simulink model "closed_loop"  (R2019a)
settings: Solver=FixedStepAuto  StartTime=0.0  StopTime=20  FixedStep=1/100  RelTol=1e-3  AbsTol=1e-3
model workspace: external: MAT-File params.mat (data not in the file)
values from neighbouring files (symbols this model uses):
  An = double(subs(A, [x;ctrl] , [x_lin; u_lin] ))    [linearization.m]
  b = 2.75E-11    (= 2.75e-11)    [linearization.m]    (also in main.m)
  Bn = double(subs(B, [x;ctrl] , [x_lin; u_lin] ))    [linearization.m]
  Cn = eye(size(x,1))    [linearization.m]
  Dn = zeros(size(x,1),4)    [linearization.m]
  g = 9.81    [linearization.m]    (also in main.m)
  k = 1E-9    (= 1e-09)    [linearization.m]    (also in main.m)
  m = 0.027    [linearization.m]    (also in main.m)
  ref_base_thrust = 0    [main.m]
  ref_roll_pitch_yawrate = [0 0 0]'    [main.m]
  u_lin = repmat(0.027*g/4, [4 1])    [main.m]
  x0 = [0 0 0  0 0 0  deg2rad(20) deg2rad(20) deg2rad(0) 0 0 0]'    [main.m]
  x_lin = zeros(12,1)    [main.m]
libraries: nesl_utility x9
settings Model: Creator=Jocke  LastModifiedBy=lucas
settings SolverCC: AutoScaleAbsTol=off
settings DataIOCC: ReturnWorkspaceOutputs=off
settings OptimizationCC: UseDivisionForNetSlopeComputation=on
settings DebuggingCC: ArithmeticOperatorsInVariantConditions=warning
settings SFSimCC: SimUseLocalCustomCode=off
settings RTWCC: RTWUseLocalCustomCode=off
settings CodeAppCC: StateflowObjectComments=on
settings SimscapeCC: SimscapeNormalizeSystem=off  SimscapeLogType=all  SimscapeLogDataHistory=10000

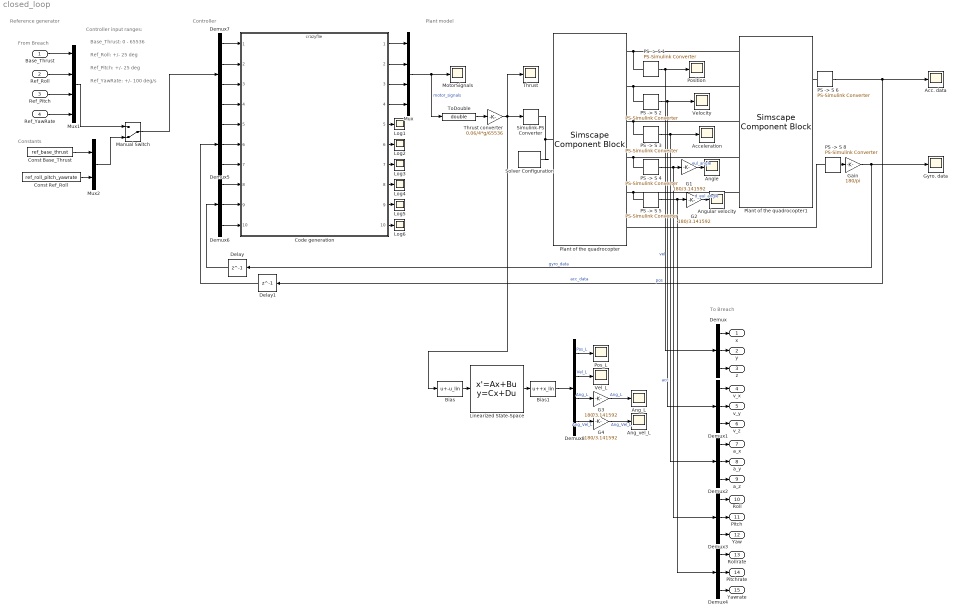
== system closed_loop ==
  note: To Breach
  note: From Breach
  note: Plant model
  note: Controller
  note: Constants
  note: Reference generator
  note: Ref_Roll: +/- 25 deg
  note: Base_Thrust: 0 - 65536
  note: Ref_Pitch: +/- 25 deg
  note: Ref_YawRate: +/- 100 deg/s
  note: Controller input ranges:
  Base_Thrust : Inport  OutDataTypeStr=double
  Ref_Roll : Inport  Port=2  OutDataTypeStr=double
  Ref_Pitch : Inport  Port=3  OutDataTypeStr=double
  Ref_YawRate : Inport  Port=4  OutDataTypeStr=double
  Acc. data : Scope
  Acceleration : Scope
  Ang_L : Scope
  Ang_vel_L : Scope
  Angle : Scope
  Angular velocity : Scope
  Bias : Bias  Bias=-u_lin
  Bias1 : Bias  Bias=+x_lin
  Code generation : ModelReference  ModelNameDialog=crazyflie.slx  SimulationMode=Normal  ModelReferenceVersion=1.283
  Const Base_Thrust : Constant  Value=ref_base_thrust
  Const Ref_Roll : Constant  Value=ref_roll_pitch_yawrate
  Delay : Delay  DelayLength=1
  Delay1 : Delay  DelayLength=1
  Demux{,1..6} (7 alike) : Demux  Outputs=3
  Demux7 : Demux
  Demux8 : Demux
  G{1..4} (4 alike) : Gain  Gain=180/3.141592
  Gain : Gain  Gain=180/pi
  Gyro. data : Scope
  Linearized State-Space : StateSpace  A=An  B=Bn  C=Cn  D=Dn  InitialCondition=x0
  Log{1..6} (6 alike) : Scope
  Manual Switch : ManualSwitch  CurrentSetting=0
  MotorSignals : Scope
  Mux : Mux
  Mux1 : Mux
  Mux2 : Mux  Inputs=2
  PS -> S {1..6,8} (7 alike) : nesl_utility/PS-Simulink Converter  PhysicalDomain=network_engine_domain  SubClassName=ps_output  LeftPortType=input  RightPortType=output  PseudoPeriodic=off  Frequencies=[]  Unit=1  AffineConversion=off
  Plant of the quadrocopter : SimscapeComponentBlock  SourceFile=plant  ComponentPath=plant  ComponentVariants=plant  ComponentVariantNames=plant  ClassName=plant  SchemaVersion=1  m=m kg  g=g m/s^2  d=d m  k=k s^2*N/rad^2  b=b N*m/(rad/s)^2  x0=x0
      settings: CopyFcn=simscape.engine.sli.internal.componentblockcallback(gcbh,'COPY')  PreCopyFcn=simscape.engine.sli.internal.componentblockcallback(gcbh,'PRECOPY')  PreDeleteFcn=simscape.engine.sli.internal.componentblockcallback(gcbh,'PREDELETE')
      mask Type: Plant of quadrocopter
  Plant of the quadrocopter1 : SimscapeComponentBlock  SourceFile=sensors  ComponentPath=sensors  ComponentVariants=sensors  ComponentVariantNames=sensors  ClassName=sensors  SchemaVersion=1
      settings: CopyFcn=simscape.engine.sli.internal.componentblockcallback(gcbh,'COPY')  PreCopyFcn=simscape.engine.sli.internal.componentblockcallback(gcbh,'PRECOPY')  PreDeleteFcn=simscape.engine.sli.internal.componentblockcallback(gcbh,'PREDELETE')
      mask Type: Plant of quadrocopter
  Pos_L : Scope
  Position : Scope
  Simulink-PS Converter : nesl_utility/Simulink-PS Converter  PhysicalDomain=network_engine_domain  SubClassName=ps_input  LeftPortType=input  RightPortType=output  PseudoPeriodic=off  Frequencies=[]  NoiseDistribution=none  NoiseParameters=[]  Unit=1  AffineConversion=off  FilteringAndDerivatives=zero  SimscapeFilterOrder=1  InputFilterTimeConstant=0.001  UdotUserProvided=1
  Solver Configuration : nesl_utility/Solver Configuration  PhysicalDomain=network_engine_domain  SubClassName=solver  LeftPortType=input  RightPortType=generic  Tones=[]  Harmonics=[]  SimulateNoise=off  Profile=off  UseLocalSampling=off  EnableSwitchedLinearOptims=on  FrequencyDomain=off  UseCCode=off  RelTol=0.001  AbsTol=1e-06  MinStep=1e-09  ToWorkspace=off  RevertToSquareIcSolve=off  NumHomotopyIterations=100  PhasorMode=off  PhasorModeNumHarmonics=1  DoDC=off  ResidualTolerance=1e-09  UseLocalSolver=off  LocalSolverChoice=NE_BACKWARD_EULER_ADVANCER  LocalSolverSampleTime=0.001  DoFixedCost=off  MaxNonlinIter=3  MaxModeIter=2  LinearAlgebra=Sparse  EquationFormulation=NE_TIME_EF  DelaysMemoryBudget=1024  AutomaticFiltering=on  FilteringTimeConstant=0.001  PartitionStorageMethod=AS_NEEDED  PartitionMemoryBudget=1024  PartitionMethod=FAST
  Thrust : Scope
  Thrust converter : Gain  Gain=0.06/4*g/65536
  ToDouble : DataTypeConversion  OutDataTypeStr=double  RndMeth=Round  SaturateOnIntegerOverflow=on
  Vel_L : Scope
  Velocity : Scope
  x : Outport
  y : Outport  Port=2
  z : Outport  Port=3
  v_x : Outport  Port=4
  v_y : Outport  Port=5
  v_z : Outport  Port=6
  a_x : Outport  Port=7
  a_y : Outport  Port=8
  a_z : Outport  Port=9
  Roll : Outport  Port=10
  Pitch : Outport  Port=11
  Yaw : Outport  Port=12
  Rollrate : Outport  Port=13
  Pitchrate : Outport  Port=14
  Yawrate : Outport  Port=15
  wires:
  Code generation/1 -> Mux/1
  Code generation/4 -> Mux/4
  Code generation/3 -> Mux/3
  Code generation/2 -> Mux/2
  Demux/1 -> x/1
  Demux/2 -> y/1
  Demux/3 -> z/1
  Demux1/1 -> v_x/1
  Demux1/2 -> v_y/1
  Demux1/3 -> v_z/1
  Demux3/1 -> Roll/1
  Demux3/2 -> Pitch/1
  Demux3/3 -> Yaw/1
  Demux4/1 -> Rollrate/1
  Demux4/2 -> Pitchrate/1
  Demux4/3 -> Yawrate/1
  Demux2/1 -> a_x/1
  Demux2/2 -> a_y/1
  Demux2/3 -> a_z/1
  Demux5/1 -> Code generation/5
  Demux5/2 -> Code generation/6
  Demux5/3 -> Code generation/7
  Demux6/1 -> Code generation/8
  Demux6/2 -> Code generation/9
  Demux6/3 -> Code generation/10
  Gain/1 -> Delay/1, Gyro. data/1  "gyro_data"
  "PS -> S 6"/1 -> Acc. data/1, Delay1/1  "acc_data"
  Code generation/5 -> Log1/1
  Code generation/6 -> Log2/1
  Code generation/7 -> Log3/1
  Code generation/8 -> Log4/1
  Code generation/9 -> Log5/1
  Code generation/10 -> Log6/1
  Base_Thrust/1 -> Mux1/1
  Ref_Roll/1 -> Mux1/2
  Ref_Pitch/1 -> Mux1/3
  Ref_YawRate/1 -> Mux1/4
  Mux1/1 -> Manual Switch/1
  Const Base_Thrust/1 -> Mux2/1
  Const Ref_Roll/1 -> Mux2/2
  Manual Switch/1 -> Demux7/1
  Demux7/1 -> Code generation/1
  Demux7/2 -> Code generation/2
  Demux7/3 -> Code generation/3
  Demux7/4 -> Code generation/4
  G1/1 -> Angle/1  "eul_angle"
  G2/1 -> Angular velocity/1  "d_eul_angle"
  ToDouble/1 -> Thrust converter/1
  Thrust converter/1 -> Bias/1, Thrust/1, Simulink-PS Converter/1
  "PS -> S 1"/1 -> Demux/1, Position/1  "pos"
  "PS -> S 5"/1 -> Demux4/1, G2/1
  "PS -> S 4"/1 -> Demux3/1, G1/1
  "PS -> S 3"/1 -> Demux2/1, Acceleration/1  "acc"
  "PS -> S 2"/1 -> Demux1/1, Velocity/1  "vel"
  Mux2/1 -> Manual Switch/2
  Mux/1 -> MotorSignals/1, ToDouble/1  "motor_signals"
  Delay/1 -> Demux6/1
  Delay1/1 -> Demux5/1
  Bias/1 -> Linearized State-Space/1
  G3/1 -> Ang_L/1  "Ang_L"
  Linearized State-Space/1 -> Bias1/1
  Demux8/2 -> Vel_L/1  "Vel_L"
  Demux8/1 -> Pos_L/1  "Pos_L"
  Demux8/3 -> G3/1  "Ang_L"
  Demux8/4 -> G4/1  "Ang_Vel_L"
  Bias1/1 -> Demux8/1
  G4/1 -> Ang_vel_L/1  "Ang_Vel_L"
  "PS -> S 8"/1 -> Gain/1
  connections:
  Simulink-PS Converter/RConn1 -- Solver Configuration/RConn1 -- Plant of the quadrocopter/LConn1
  Plant of the quadrocopter1/LConn1 -- "PS -> S 1"/LConn1 -- Plant of the quadrocopter/RConn1
  Plant of the quadrocopter1/LConn2 -- "PS -> S 2"/LConn1 -- Plant of the quadrocopter/RConn2
  Plant of the quadrocopter1/LConn3 -- "PS -> S 3"/LConn1 -- Plant of the quadrocopter/RConn3
  Plant of the quadrocopter1/LConn4 -- "PS -> S 4"/LConn1 -- Plant of the quadrocopter/RConn4
  Plant of the quadrocopter1/LConn5 -- "PS -> S 5"/LConn1 -- Plant of the quadrocopter/RConn5
  Plant of the quadrocopter1/RConn1 -- "PS -> S 6"/LConn1
  "PS -> S 8"/LConn1 -- Plant of the quadrocopter/RConn6
